simulink model "Simulink_Lab02_TCA1"  (R2026a)
settings: Solver=VariableStepAuto
settings Model: Creator=NITRO V15  LastModifiedBy=NITRO V15

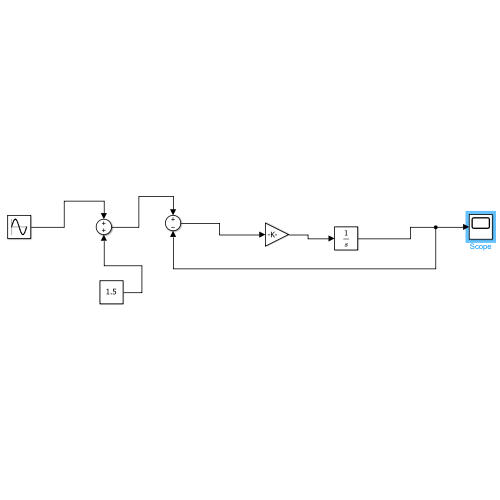
[thumbnail: Simulink's stored preview of the top-level diagram]
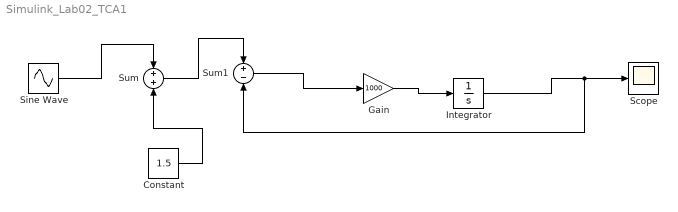
== system Simulink_Lab02_TCA1 ==
  Constant : Constant  Value=1.5
  Gain : Gain  Gain=1000
  Integrator : Integrator
  Scope : Scope
      settings: ActiveDisplayYMinimum=-0.31215443161277107  ActiveDisplayYMaximum=2.80938988451494
  Sine Wave : Sin  Frequency=2*pi*10  SampleTime=0
  Sum : Sum
  Sum1 : Sum  Inputs=+-
  wires:
  Sine Wave/1 -> Sum/1
  Constant/1 -> Sum/2
  Sum/1 -> Sum1/1
  Sum1/1 -> Gain/1
  Gain/1 -> Integrator/1
  Integrator/1 -> Sum1/2, Scope/1
